simulink model "GliderYawResponseModel"  (R2013a)
settings: Solver=ode3  StartTime=0.0  StopTime=80  FixedStep=1e-2  RelTol=1e-3
libraries: simulink x4
settings Model: Creator=user  LastModifiedBy=user

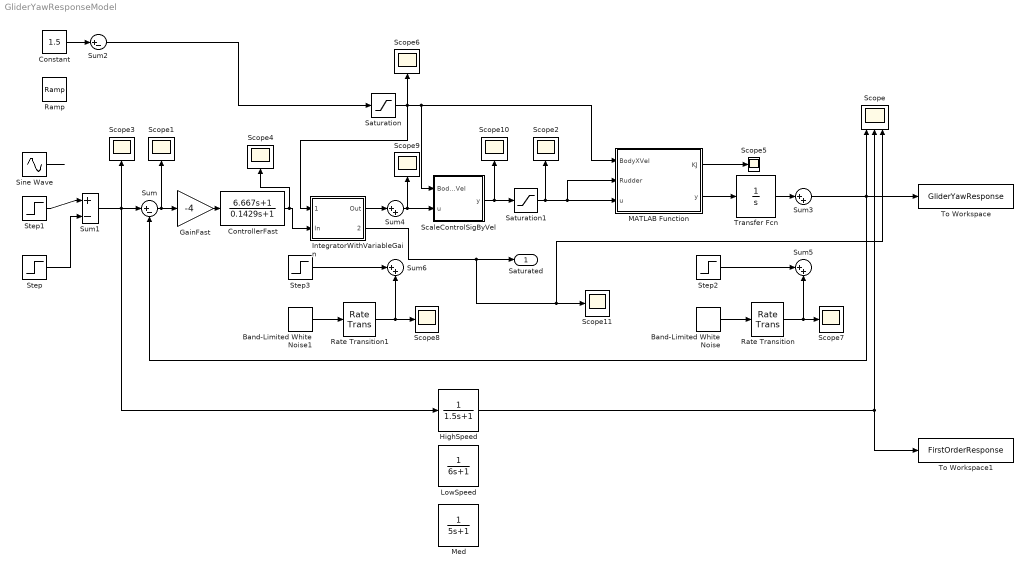
== system GliderYawResponseModel ==
  Band-Limited White Noise : simulink/Sources/Band-Limited White Noise  Cov=[0.0000000]  Ts=0.01  seed=[23341]
  Band-Limited White Noise1 : simulink/Sources/Band-Limited White Noise  Cov=[0.000]  Ts=0.01  seed=[23341]
  Constant : Constant  Value=1.5
  ControllerFast : TransferFcn  Numerator=[6.667 1]  Denominator=[0.1429 1]
  GainFast : Gain  Gain=-4
  HighSpeed : TransferFcn  Denominator=[1.5 1]
  IntegratorWithVariableGain : Subsystem
  LowSpeed : TransferFcn  Denominator=[6 1]
  MATLAB Function : MATLAB Function  TreatAsAtomicUnit=on
  Med : TransferFcn  Denominator=[5 1]
  Ramp : simulink/Sources/Ramp  slope=0.005  start=5  X0=0
  Rate Transition : RateTransition
  Rate Transition1 : RateTransition
  Saturation : Saturate  UpperLimit=1.5  LowerLimit=0.1
  Saturation1 : Saturate  UpperLimit=pi/18*5  LowerLimit=-pi/18*5
  ScaleControlSigByVel : MATLAB Function  TreatAsAtomicUnit=on
  Scope : Scope  NumInputPorts=3
      settings: TimeRange=60  YMin=0~-5~-5  YMax=0.225~5~5
  Scope{1..11} (11 alike) : Scope
      Scope10 settings: TimeRange=120  YMin=-1  YMax=0.4000000000000001  SaveName=ScopeData10
      Scope11 settings: YMin=-1.25  YMax=1.25  SaveName=ScopeData11
      Scope2 settings: TimeRange=120  YMin=-1  YMax=0.4000000000000001  SaveName=ScopeData2
      Scope3 settings: SaveName=ScopeData3
      Scope4 settings: YMax=1  SaveName=ScopeData4
      Scope5 settings: SaveName=ScopeData5
      Scope6 settings: SaveName=ScopeData6
      Scope7 settings: SaveName=ScopeData7
      Scope8 settings: YMin=-1.25  YMax=1.25  SaveName=ScopeData8
      Scope9 settings: SaveName=ScopeData9
  Sine Wave : Sin  Amplitude=0.01  Frequency=0.2  SampleTime=0
  Step : Step  Time=7  After=0  SampleTime=0
  Step1 : Step  Time=5  After=0.05  SampleTime=0
  Step2 : Step  Time=40  After=0.00  SampleTime=0
  Step3 : Step  Time=80  After=0.0  SampleTime=0
  Sum : Sum  Inputs=|+-
  Sum1 : Sum  Inputs=|+-
  Sum2 : Sum  Inputs=|+-
  Sum3 : Sum  Inputs=|++
  Sum4 : Sum  Inputs=|++
  Sum5 : Sum  Inputs=++|
  Sum6 : Sum  Inputs=++|
  To Workspace : ToWorkspace  VariableName=GliderYawResponse  SampleTime=-1
  To Workspace1 : ToWorkspace  VariableName=FirstOrderResponse  SampleTime=-1
  Transfer Fcn : TransferFcn  Denominator=[1 0]
  Saturated : Outport
  wires:
  Step3/1 -> Sum6/1
  Band-Limited White Noise1/1 -> Rate Transition1/1
  IntegratorWithVariableGain/2(Saturated) -> Scope/3, Scope11/1, Saturated/1
  ControllerFast/1 -> IntegratorWithVariableGain/2(In), Scope4/1
  MATLAB Function/1(KJ) -> Scope5/1
  Rate Transition1/1 -> Scope8/1, Sum6/2
  Sum1/1 -> HighSpeed/1, Scope3/1, Sum/1
  Sum/1 -> GainFast/1, Scope1/1
  MATLAB Function/2(y) -> Transfer Fcn/1
  Sum2/1 -> Saturation/1
  Rate Transition/1 -> Sum5/2, Scope7/1
  Transfer Fcn/1 -> Sum3/1
  GainFast/1 -> ControllerFast/1
  Band-Limited White Noise/1 -> Rate Transition/1
  Sum4/1 -> Scope9/1, ScaleControlSigByVel/2(u)
  ScaleControlSigByVel/1(y) -> Saturation1/1, Scope10/1
  Step2/1 -> Sum5/1
  Saturation/1 -> IntegratorWithVariableGain/1(BodyXVel), MATLAB Function/1(BodyXVel), ScaleControlSigByVel/1(BodyXVel), Scope6/1
  IntegratorWithVariableGain/1(Out) -> Sum4/1
  Saturation1/1 -> MATLAB Function/2(Rudder), MATLAB Function/3(u), Scope2/1
  Sum3/1 -> To Workspace/1, Scope/1, Sum/2
  Step1/1 -> Sum1/1
  Step/1 -> Sum1/2
  Constant/1 -> Sum2/1
  HighSpeed/1 -> To Workspace1/1, Scope/2
  Sine Wave/1 -> ?

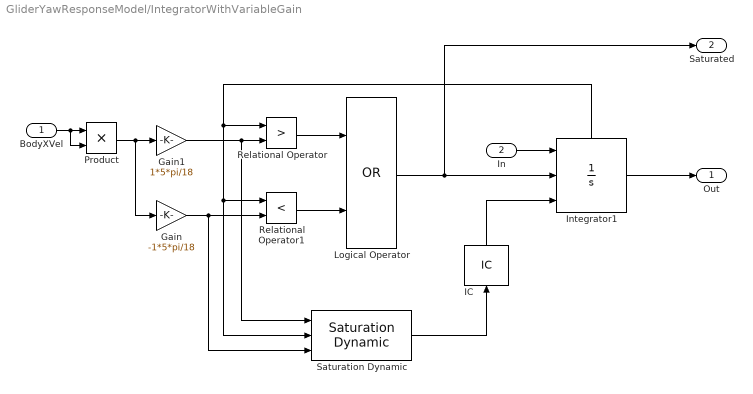
== system GliderYawResponseModel/IntegratorWithVariableGain ==
  BodyXVel : Inport
  In : Inport  Port=2
  Gain : Gain  Gain=-1*5*pi/18
  Gain1 : Gain  Gain=1*5*pi/18
  IC : InitialCondition  Value=0
  Integrator1 : Integrator  ExternalReset=level  InitialConditionSource=external  UpperSaturationLimit=5*pi/8  LowerSaturationLimit=-5*pi/8  ShowStatePort=on
  Logical Operator : Logic  Operator=OR  AllPortsSameDT=off  OutDataTypeStr=boolean
  Product : Product
  Relational Operator : RelationalOperator  Operator=>  OutDataTypeStr=boolean
  Relational Operator1 : RelationalOperator  Operator=<  OutDataTypeStr=boolean
  Saturation Dynamic : simulink/Discontinuities/Saturation Dynamic  OutMin=[]  OutMax=[]  OutDataTypeStr=Inherit: Same as second input  OutDataType=fixdt(1, 16)  OutScaling=2^-10  DoSatur=off
  Out : Outport
  Saturated : Outport  Port=2
  wires:
  In/1 -> Integrator1/1
  Integrator1/1 -> Out/1
  Relational Operator/1 -> Logical Operator/1
  Relational Operator1/1 -> Logical Operator/2
  Integrator1/State -> Relational Operator/1, Saturation Dynamic/2, Relational Operator1/1
  Gain1/1 -> Saturation Dynamic/1, Relational Operator/2
  Gain/1 -> Saturation Dynamic/3, Relational Operator1/2
  Logical Operator/1 -> Saturated/1, Integrator1/2
  Saturation Dynamic/1 -> IC/1
  IC/1 -> Integrator1/3
  BodyXVel/1 -> Product/2, Product/1
  Product/1 -> Gain/1, Gain1/1

== matlab function GliderYawResponseModel/MATLAB Function ==
  data: KJ output; BodyXVel input; Rudder input; u input; y output
function [KJ,y] = fcn(BodyXVel,Rudder,u)
%#codegen
RudderM = abs(Rudder);

% % First set of tests, long averaging time
% p00 =   0.0005488;
% p10 =    -0.03384;
% p01 =     0.02284;
% p20 =      0.1475;
% p11 =     -0.1365;
% p02 =    -0.02259;
% p30 =     -0.1176;
% p21 =     0.08015;
% p12 =    -0.04739;
% 
% 
% KJ = p00 + p10*RudderM + p01*BodyXVel + p20*RudderM^2 +...
%     p11*RudderM*BodyXVel + p02*BodyXVel^2 + p30*RudderM^3 +...
%     p21*RudderM^2*BodyXVel + p12*RudderM*BodyXVel^2;

% Second set of tests, short averaging time
p00 =    0.001019;
p10 =    -0.03252;
p01 =    0.007799;
p20 =      0.1448;
p11 =    -0.08634;
p02 =   -0.008142;
p30 =     -0.1309;
p21 =     0.09769;
p12 =     -0.1151;

KJ = p00 + p10*RudderM + p01*BodyXVel + p20*RudderM^2 + p11*RudderM*BodyXVel + p02*BodyXVel^2 ...
    + p30*RudderM^3 + p21*RudderM^2*BodyXVel + p12*RudderM*BodyXVel^2;

if KJ>-0.001
    KJ = -0.001;
end

y = KJ*u;

== matlab function GliderYawResponseModel/ScaleControlSigByVel ==
  data: BodyXVel input; u input; y output
function y = fcn(BodyXVel,u)
%#codegen

y = u/(BodyXVel^2);
